simulink model "duffing_simulation"  (R2018a)
settings: Solver=ode23  StartTime=0.0  StopTime=1000  RelTol=1e-3
values from neighbouring files (symbols this model uses):
  gamma = 1/(4*Q)    (= 0.0025)    [sim_run.m]
  T = sim.get('T')    [sim_run.m]
  zeta = 1/(2*Q)    (= 0.005)    [sim_run.m]
settings Model: Creator=Shay  LastModifiedBy=Shay

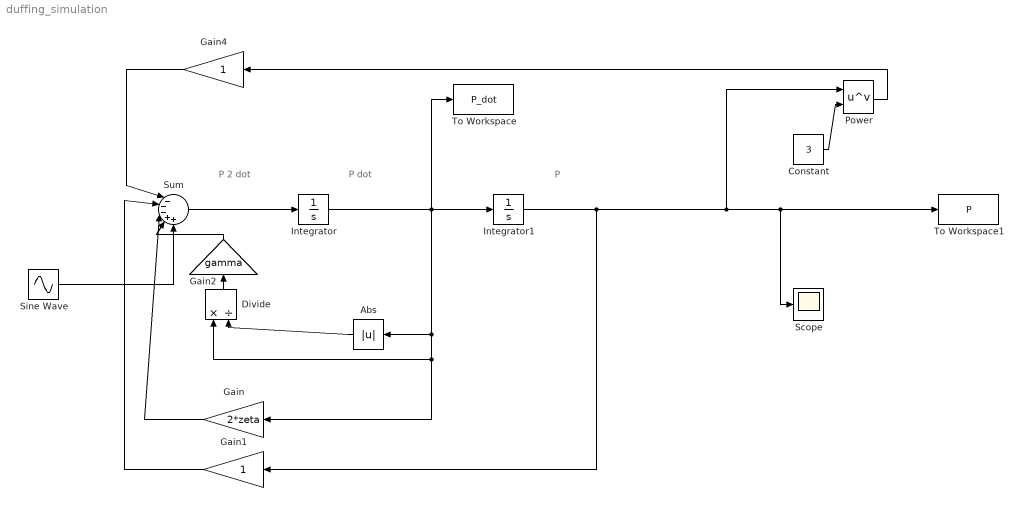
== system duffing_simulation ==
  note: P 2 dot
  note: P dot
  note: P
  Abs : Abs  ZeroCross=off
  Constant : Constant  Value=3
  Divide : Product  Inputs=*/
  Gain : Gain  Gain=2*zeta
  Gain1 : Gain
  Gain2 : Gain  Gain=gamma
  Gain4 : Gain
  Integrator : Integrator  InitialCondition=1
  Integrator1 : Integrator  InitialCondition=1
  Power : Math  Operator=pow  SaturateOnIntegerOverflow=on
  Scope : Scope
  Sine Wave : Sin  Phase=pi/2  SampleTime=T
  Sum : Sum  Inputs=|---++
  To Workspace : ToWorkspace  VariableName=P_dot  SampleTime=-1
  To Workspace1 : ToWorkspace  VariableName=P  SampleTime=-1
  wires:
  Sum/1 -> Integrator/1
  Integrator/1 -> Gain/1, Divide/1, Abs/1, Integrator1/1, To Workspace/1
  Constant/1 -> Power/2
  Integrator1/1 -> Gain1/1, Scope/1, To Workspace1/1, Power/1
  Power/1 -> Gain4/1
  Gain4/1 -> Sum/1
  Gain/1 -> Sum/3
  Gain1/1 -> Sum/2
  Abs/1 -> Divide/2
  Divide/1 -> Gain2/1
  Gain2/1 -> Sum/4
  Sine Wave/1 -> Sum/5
